simulink model "Lab4_ReplayCompare"  (R2025b)
settings: Solver=ode3  StartTime=0.0  StopTime=replay_Tend  FixedStep=Ts/4  RelTol=1e-3
PreLoadFcn:
  | if ~exist('replay_source','var'), which_log='VF'; else which_log='VF'; end; prep_replay_lab4(which_log);
settings Model: Creator=Lubin Kerhuel  LastModifiedBy=Lubin Kerhuel
settings DataIOCC: ReturnWorkspaceOutputs=off
settings OptimizationCC: LifeSpan=1

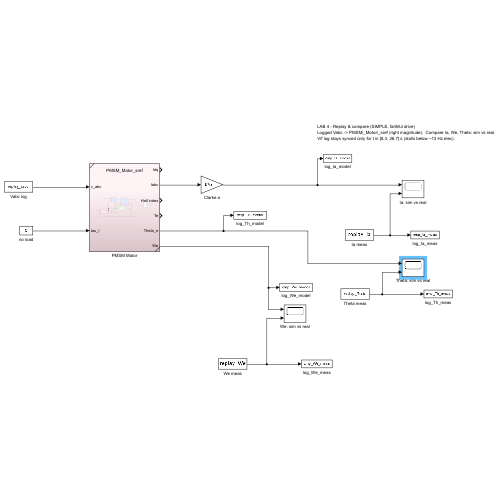
[thumbnail: Simulink's stored preview of the top-level diagram]
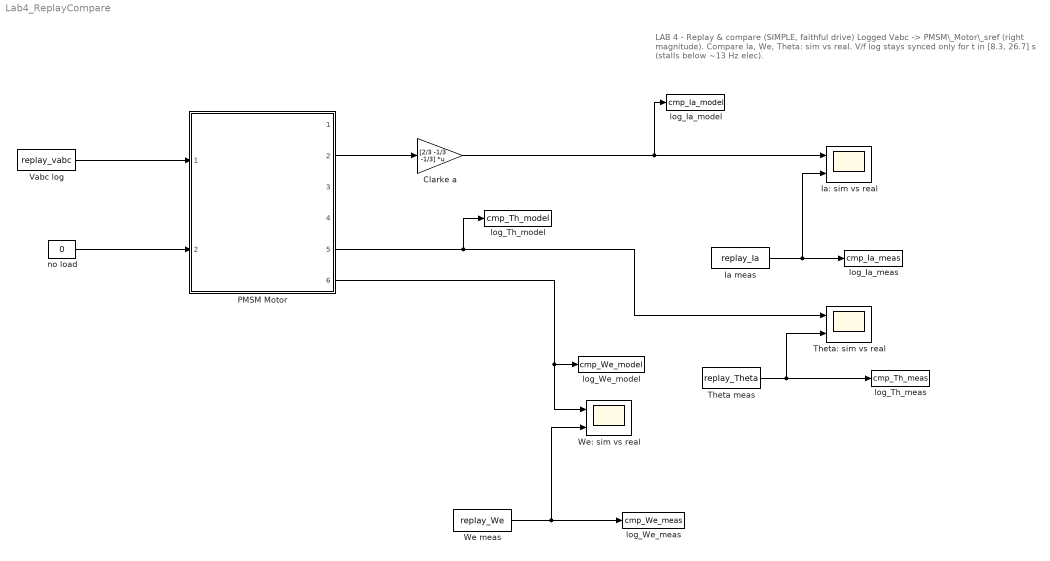
== system Lab4_ReplayCompare ==
  note: LAB 4 - Replay & compare (SIMPLE, faithful drive)
      | Logged Vabc -> PMSM\_Motor\_sref (right magnitude).  Compare Ia, We, Theta: sim vs real.
      | V/f log stays synced only for t in [8.3, 26.7] s (stalls below ~13 Hz elec).
  Clarke a : Gain  Gain=[2/3 -1/3 -1/3]  Multiplication=Matrix(K*u)
  Ia meas : FromWorkspace  VariableName=replay_Ia  OutputAfterFinalValue=Holding final value
  Ia: sim vs real : Scope  NumInputPorts=2
      settings: ActiveDisplayYMinimum=-25.745222182083133  ActiveDisplayYMaximum=11.26599963874817
  PMSM Motor : Subsystem  ReferencedSubsystem=PMSM_Motor_sref
  Theta meas : FromWorkspace  VariableName=replay_Theta  OutputAfterFinalValue=Holding final value
  Theta: sim vs real : Scope  NumInputPorts=2
      settings: ActiveDisplayYMinimum=-0.15228849345667594  ActiveDisplayYMaximum=6.4611387785664149
  Vabc log : FromWorkspace  VariableName=replay_vabc  OutputAfterFinalValue=Holding final value
  We meas : FromWorkspace  VariableName=replay_We  OutputAfterFinalValue=Holding final value
  We: sim vs real : Scope  NumInputPorts=2
      settings: ActiveDisplayYMinimum=-36.461671226193204  ActiveDisplayYMaximum=354.250322245605
  log_Ia_meas : ToWorkspace  VariableName=cmp_Ia_meas  SaveFormat=Timeseries  SampleTime=-1
  log_Ia_model : ToWorkspace  VariableName=cmp_Ia_model  SaveFormat=Timeseries  SampleTime=-1
  log_Th_meas : ToWorkspace  VariableName=cmp_Th_meas  SaveFormat=Timeseries  SampleTime=-1
  log_Th_model : ToWorkspace  VariableName=cmp_Th_model  SaveFormat=Timeseries  SampleTime=-1
  log_We_meas : ToWorkspace  VariableName=cmp_We_meas  SaveFormat=Timeseries  SampleTime=-1
  log_We_model : ToWorkspace  VariableName=cmp_We_model  SaveFormat=Timeseries  SampleTime=-1
  no load : Constant  Value=0
  wires:
  We meas/1 -> We: sim vs real/2, log_We_meas/1
  Theta meas/1 -> log_Th_meas/1, Theta: sim vs real/2
  PMSM Motor/6 -> We: sim vs real/1, log_We_model/1
  PMSM Motor/2 -> Clarke a/1
  no load/1 -> PMSM Motor/2
  Ia meas/1 -> Ia: sim vs real/2, log_Ia_meas/1
  Vabc log/1 -> PMSM Motor/1
  PMSM Motor/5 -> Theta: sim vs real/1, log_Th_model/1
  Clarke a/1 -> Ia: sim vs real/1, log_Ia_model/1
